simulink library "xps_library"  (Simulink 8.2)
settings: Solver=ode45  SolverMode=SingleTasking  StartTime=0.0  StopTime=10.0  RelTol=1e-3
undefined symbols (not defined in the file): sys_clk
libraries: xbsIndex_r4 x865, dspsigops x81, simulink x68, casper_library_flow_control x68, xps_library x25, casper_library_misc x4
(part 4 of 10)

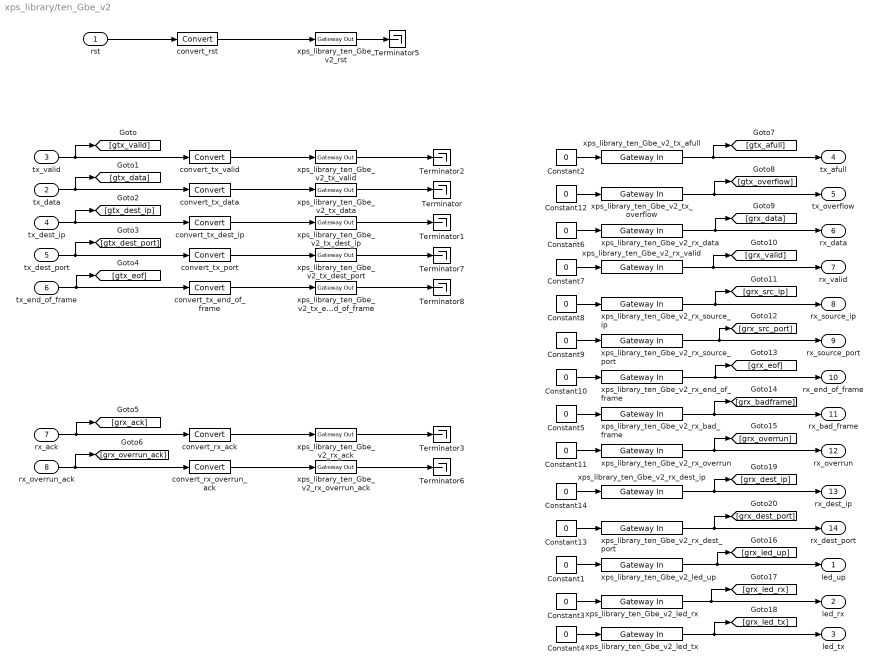
== system xps_library/ten_Gbe_v2 ==
  rst : Inport
  tx_data : Inport  Port=2
  tx_valid : Inport  Port=3
  tx_dest_ip : Inport  Port=4
  tx_dest_port : Inport  Port=5
  tx_end_of_frame : Inport  Port=6
  rx_ack : Inport  Port=7
  rx_overrun_ack : Inport  Port=8
  Constant{1..14} (14 alike) : Constant  Value=0
  Terminator{,1..3,5..8} (8 alike) : Terminator
  convert_rst : xbsIndex_r4/Convert  gui_display_data_type=Fixed-point  arith_type=Boolean  n_bits=64  bin_pt=0  float_type=Single  exp_bits=8  fraction_bits=24  quantization=Truncate  overflow=Wrap  en=off  latency=0  dbl_ovrd=off  pipeline=off  block_type=convert
      settings: xl_area=[0, 0, 0, 0, 0, 0, 0]
  convert_rx_ack : xbsIndex_r4/Convert  gui_display_data_type=Fixed-point  arith_type=Boolean  n_bits=64  bin_pt=0  float_type=Single  exp_bits=8  fraction_bits=24  quantization=Truncate  overflow=Wrap  en=off  latency=0  dbl_ovrd=off  pipeline=off  block_type=convert
      settings: xl_area=[0, 0, 0, 0, 0, 0, 0]
  convert_rx_overrun_ack : xbsIndex_r4/Convert  gui_display_data_type=Fixed-point  arith_type=Boolean  n_bits=64  bin_pt=0  float_type=Single  exp_bits=8  fraction_bits=24  quantization=Truncate  overflow=Wrap  en=off  latency=0  dbl_ovrd=off  pipeline=off  block_type=convert
      settings: xl_area=[0, 0, 0, 0, 0, 0, 0]
  convert_tx_data : xbsIndex_r4/Convert  gui_display_data_type=Fixed-point  arith_type=Unsigned  n_bits=64  bin_pt=0  float_type=Single  exp_bits=8  fraction_bits=24  quantization=Truncate  overflow=Wrap  en=off  latency=0  dbl_ovrd=off  pipeline=off  block_type=convert
      settings: xl_area=[0, 0, 0, 0, 0, 0, 0]
  convert_tx_dest_ip : xbsIndex_r4/Convert  gui_display_data_type=Fixed-point  arith_type=Unsigned  n_bits=32  bin_pt=0  float_type=Single  exp_bits=8  fraction_bits=24  quantization=Truncate  overflow=Wrap  en=off  latency=0  dbl_ovrd=off  pipeline=off  block_type=convert
      settings: xl_area=[0, 0, 0, 0, 0, 0, 0]
  convert_tx_end_of_frame : xbsIndex_r4/Convert  gui_display_data_type=Fixed-point  arith_type=Boolean  n_bits=1  bin_pt=0  float_type=Single  exp_bits=8  fraction_bits=24  quantization=Truncate  overflow=Wrap  en=off  latency=0  dbl_ovrd=off  pipeline=off  block_type=convert
      settings: xl_area=[0, 0, 0, 0, 0, 0, 0]
  convert_tx_port : xbsIndex_r4/Convert  gui_display_data_type=Fixed-point  arith_type=Unsigned  n_bits=16  bin_pt=0  float_type=Single  exp_bits=8  fraction_bits=24  quantization=Truncate  overflow=Wrap  en=off  latency=0  dbl_ovrd=off  pipeline=off  block_type=convert
      settings: xl_area=[0, 0, 0, 0, 0, 0, 0]
  convert_tx_valid : xbsIndex_r4/Convert  gui_display_data_type=Fixed-point  arith_type=Boolean  n_bits=1  bin_pt=0  float_type=Single  exp_bits=8  fraction_bits=24  quantization=Truncate  overflow=Wrap  en=off  latency=0  dbl_ovrd=off  pipeline=off  block_type=convert
      settings: xl_area=[0, 0, 0, 0, 0, 0, 0]
  xps_library_ten_Gbe_v2_led_rx : xbsIndex_r4/Gateway In  gui_display_data_type=Fixed-point  arith_type=Boolean  n_bits=1  bin_pt=0  preci_type=Single  exp_width=8  frac_width=24  quantization=Truncate  overflow=Wrap  period=1  dbl_ovrd=off  timing_constraint=None  locs_specified=off  LOCs={}  UseAsADC=off  ADCChannel='1'  inherit_from_input=off  hdl_port=on  block_type=gatewayin
      settings: infoedit="Gateway in block.  Converts inputs of type Simulink integer, double and fixed point to  Xilinx fixed point type.<P><P>Hardware notes:  In hardware these blocks become top level input ports."  xl_area=[0, 0, 0, 0, 0, 0, 0]
  xps_library_ten_Gbe_v2_led_tx : xbsIndex_r4/Gateway In  gui_display_data_type=Fixed-point  arith_type=Boolean  n_bits=1  bin_pt=0  preci_type=Single  exp_width=8  frac_width=24  quantization=Truncate  overflow=Wrap  period=1  dbl_ovrd=off  timing_constraint=None  locs_specified=off  LOCs={}  UseAsADC=off  ADCChannel='1'  inherit_from_input=off  hdl_port=on  block_type=gatewayin
      settings: infoedit="Gateway in block.  Converts inputs of type Simulink integer, double and fixed point to  Xilinx fixed point type.<P><P>Hardware notes:  In hardware these blocks become top level input ports."  xl_area=[0, 0, 0, 0, 0, 0, 0]
  xps_library_ten_Gbe_v2_led_up : xbsIndex_r4/Gateway In  gui_display_data_type=Fixed-point  arith_type=Boolean  n_bits=1  bin_pt=0  preci_type=Single  exp_width=8  frac_width=24  quantization=Truncate  overflow=Wrap  period=1  dbl_ovrd=off  timing_constraint=None  locs_specified=off  LOCs={}  UseAsADC=off  ADCChannel='1'  inherit_from_input=off  hdl_port=on  block_type=gatewayin
      settings: infoedit="Gateway in block.  Converts inputs of type Simulink integer, double and fixed point to  Xilinx fixed point type.<P><P>Hardware notes:  In hardware these blocks become top level input ports."  xl_area=[0, 0, 0, 0, 0, 0, 0]
  xps_library_ten_Gbe_v2_rst : xbsIndex_r4/Gateway Out  inherit_from_input=off  hdl_port=on  timing_constraint=None  locs_specified=off  LOCs={}  UseAsDAC=off  DACChannel='1'  block_type=gatewayout
      settings: infoedit="Gateway out block.  Converts Xilinx fixed point inputs into ouputs of type Simulink integer, double, or fixed point.<P><P>Hardware notes:  In hardware these blocks become top level output ports or are discarded, depending on how they are configured."  xl_area=[0, 0, 0, 0, 0, 0, 0]
  xps_library_ten_Gbe_v2_rx_ack : xbsIndex_r4/Gateway Out  inherit_from_input=off  hdl_port=on  timing_constraint=None  locs_specified=off  LOCs={}  UseAsDAC=off  DACChannel='1'  block_type=gatewayout
      settings: infoedit="Gateway out block.  Converts Xilinx fixed point inputs into ouputs of type Simulink integer, double, or fixed point.<P><P>Hardware notes:  In hardware these blocks become top level output ports or are discarded, depending on how they are configured."  xl_area=[0, 0, 0, 0, 0, 0, 0]
  xps_library_ten_Gbe_v2_rx_bad_frame : xbsIndex_r4/Gateway In  gui_display_data_type=Fixed-point  arith_type=Boolean  n_bits=1  bin_pt=0  preci_type=Single  exp_width=8  frac_width=24  quantization=Truncate  overflow=Wrap  period=1  dbl_ovrd=off  timing_constraint=None  locs_specified=off  LOCs={}  UseAsADC=off  ADCChannel='1'  inherit_from_input=off  hdl_port=on  block_type=gatewayin
      settings: infoedit="Gateway in block.  Converts inputs of type Simulink integer, double and fixed point to  Xilinx fixed point type.<P><P>Hardware notes:  In hardware these blocks become top level input ports."  xl_area=[0, 0, 0, 0, 0, 0, 0]
  xps_library_ten_Gbe_v2_rx_data : xbsIndex_r4/Gateway In  gui_display_data_type=Fixed-point  arith_type=Unsigned  n_bits=64  bin_pt=0  preci_type=Single  exp_width=8  frac_width=24  quantization=Truncate  overflow=Wrap  period=1  dbl_ovrd=off  timing_constraint=None  locs_specified=off  LOCs={}  UseAsADC=off  ADCChannel='1'  inherit_from_input=off  hdl_port=on  block_type=gatewayin
      settings: infoedit="Gateway in block.  Converts inputs of type Simulink integer, double and fixed point to  Xilinx fixed point type.<P><P>Hardware notes:  In hardware these blocks become top level input ports."  xl_area=[0, 0, 0, 0, 0, 0, 0]
  xps_library_ten_Gbe_v2_rx_dest_ip : xbsIndex_r4/Gateway In  gui_display_data_type=Fixed-point  arith_type=Unsigned  n_bits=32  bin_pt=0  preci_type=Single  exp_width=8  frac_width=24  quantization=Truncate  overflow=Wrap  period=1  dbl_ovrd=off  timing_constraint=None  locs_specified=off  LOCs={}  UseAsADC=off  ADCChannel='1'  inherit_from_input=off  hdl_port=on  block_type=gatewayin
      settings: xl_area=[0, 0, 0, 0, 0, 0, 0]
  xps_library_ten_Gbe_v2_rx_dest_port : xbsIndex_r4/Gateway In  gui_display_data_type=Fixed-point  arith_type=Unsigned  n_bits=16  bin_pt=0  preci_type=Single  exp_width=8  frac_width=24  quantization=Truncate  overflow=Wrap  period=1  dbl_ovrd=off  timing_constraint=None  locs_specified=off  LOCs={}  UseAsADC=off  ADCChannel='1'  inherit_from_input=off  hdl_port=on  block_type=gatewayin
      settings: xl_area=[0, 0, 0, 0, 0, 0, 0]
  xps_library_ten_Gbe_v2_rx_end_of_frame : xbsIndex_r4/Gateway In  gui_display_data_type=Fixed-point  arith_type=Boolean  n_bits=1  bin_pt=0  preci_type=Single  exp_width=8  frac_width=24  quantization=Truncate  overflow=Wrap  period=1  dbl_ovrd=off  timing_constraint=None  locs_specified=off  LOCs={}  UseAsADC=off  ADCChannel='1'  inherit_from_input=off  hdl_port=on  block_type=gatewayin
      settings: infoedit="Gateway in block.  Converts inputs of type Simulink integer, double and fixed point to  Xilinx fixed point type.<P><P>Hardware notes:  In hardware these blocks become top level input ports."  xl_area=[0, 0, 0, 0, 0, 0, 0]
  xps_library_ten_Gbe_v2_rx_overrun : xbsIndex_r4/Gateway In  gui_display_data_type=Fixed-point  arith_type=Boolean  n_bits=1  bin_pt=0  preci_type=Single  exp_width=8  frac_width=24  quantization=Truncate  overflow=Wrap  period=1  dbl_ovrd=off  timing_constraint=None  locs_specified=off  LOCs={}  UseAsADC=off  ADCChannel='1'  inherit_from_input=off  hdl_port=on  block_type=gatewayin
      settings: infoedit="Gateway in block.  Converts inputs of type Simulink integer, double and fixed point to  Xilinx fixed point type.<P><P>Hardware notes:  In hardware these blocks become top level input ports."  xl_area=[0, 0, 0, 0, 0, 0, 0]
  xps_library_ten_Gbe_v2_rx_overrun_ack : xbsIndex_r4/Gateway Out  inherit_from_input=off  hdl_port=on  timing_constraint=None  locs_specified=off  LOCs={}  UseAsDAC=off  DACChannel='1'  block_type=gatewayout
      settings: infoedit="Gateway out block.  Converts Xilinx fixed point inputs into ouputs of type Simulink integer, double, or fixed point.<P><P>Hardware notes:  In hardware these blocks become top level output ports or are discarded, depending on how they are configured."  xl_area=[0, 0, 0, 0, 0, 0, 0]
  xps_library_ten_Gbe_v2_rx_source_ip : xbsIndex_r4/Gateway In  gui_display_data_type=Fixed-point  arith_type=Unsigned  n_bits=32  bin_pt=0  preci_type=Single  exp_width=8  frac_width=24  quantization=Truncate  overflow=Wrap  period=1  dbl_ovrd=off  timing_constraint=None  locs_specified=off  LOCs={}  UseAsADC=off  ADCChannel='1'  inherit_from_input=off  hdl_port=on  block_type=gatewayin
      settings: infoedit="Gateway in block.  Converts inputs of type Simulink integer, double and fixed point to  Xilinx fixed point type.<P><P>Hardware notes:  In hardware these blocks become top level input ports."  xl_area=[0, 0, 0, 0, 0, 0, 0]
  xps_library_ten_Gbe_v2_rx_source_port : xbsIndex_r4/Gateway In  gui_display_data_type=Fixed-point  arith_type=Unsigned  n_bits=16  bin_pt=0  preci_type=Single  exp_width=8  frac_width=24  quantization=Truncate  overflow=Wrap  period=1  dbl_ovrd=off  timing_constraint=None  locs_specified=off  LOCs={}  UseAsADC=off  ADCChannel='1'  inherit_from_input=off  hdl_port=on  block_type=gatewayin
      settings: infoedit="Gateway in block.  Converts inputs of type Simulink integer, double and fixed point to  Xilinx fixed point type.<P><P>Hardware notes:  In hardware these blocks become top level input ports."  xl_area=[0, 0, 0, 0, 0, 0, 0]
  xps_library_ten_Gbe_v2_rx_valid : xbsIndex_r4/Gateway In  gui_display_data_type=Fixed-point  arith_type=Boolean  n_bits=1  bin_pt=0  preci_type=Single  exp_width=8  frac_width=24  quantization=Truncate  overflow=Wrap  period=1  dbl_ovrd=off  timing_constraint=None  locs_specified=off  LOCs={}  UseAsADC=off  ADCChannel='1'  inherit_from_input=off  hdl_port=on  block_type=gatewayin
      settings: infoedit="Gateway in block.  Converts inputs of type Simulink integer, double and fixed point to  Xilinx fixed point type.<P><P>Hardware notes:  In hardware these blocks become top level input ports."  xl_area=[0, 0, 0, 0, 0, 0, 0]
  xps_library_ten_Gbe_v2_tx_afull : xbsIndex_r4/Gateway In  gui_display_data_type=Fixed-point  arith_type=Boolean  n_bits=1  bin_pt=0  preci_type=Single  exp_width=8  frac_width=24  quantization=Truncate  overflow=Wrap  period=1  dbl_ovrd=off  timing_constraint=None  locs_specified=off  LOCs={}  UseAsADC=off  ADCChannel='1'  inherit_from_input=off  hdl_port=on  block_type=gatewayin
      settings: infoedit="Gateway in block.  Converts inputs of type Simulink integer, double and fixed point to  Xilinx fixed point type.<P><P>Hardware notes:  In hardware these blocks become top level input ports."  xl_area=[0, 0, 0, 0, 0, 0, 0]
  xps_library_ten_Gbe_v2_tx_data : xbsIndex_r4/Gateway Out  inherit_from_input=off  hdl_port=on  timing_constraint=None  locs_specified=off  LOCs={}  UseAsDAC=off  DACChannel='1'  block_type=gatewayout
      settings: infoedit="Gateway out block.  Converts Xilinx fixed point inputs into ouputs of type Simulink integer, double, or fixed point.<P><P>Hardware notes:  In hardware these blocks become top level output ports or are discarded, depending on how they are configured."  xl_area=[0, 0, 0, 0, 0, 0, 0]
  xps_library_ten_Gbe_v2_tx_dest_ip : xbsIndex_r4/Gateway Out  inherit_from_input=off  hdl_port=on  timing_constraint=None  locs_specified=off  LOCs={}  UseAsDAC=off  DACChannel='1'  block_type=gatewayout
      settings: infoedit="Gateway out block.  Converts Xilinx fixed point inputs into ouputs of type Simulink integer, double, or fixed point.<P><P>Hardware notes:  In hardware these blocks become top level output ports or are discarded, depending on how they are configured."  xl_area=[0, 0, 0, 0, 0, 0, 0]
  xps_library_ten_Gbe_v2_tx_dest_port : xbsIndex_r4/Gateway Out  inherit_from_input=off  hdl_port=on  timing_constraint=None  locs_specified=off  LOCs={}  UseAsDAC=off  DACChannel='1'  block_type=gatewayout
      settings: infoedit="Gateway out block.  Converts Xilinx fixed point inputs into ouputs of type Simulink integer, double, or fixed point.<P><P>Hardware notes:  In hardware these blocks become top level output ports or are discarded, depending on how they are configured."  xl_area=[0, 0, 0, 0, 0, 0, 0]
  xps_library_ten_Gbe_v2_tx_end_of_frame : xbsIndex_r4/Gateway Out  inherit_from_input=off  hdl_port=on  timing_constraint=None  locs_specified=off  LOCs={}  UseAsDAC=off  DACChannel='1'  block_type=gatewayout
      settings: infoedit="Gateway out block.  Converts Xilinx fixed point inputs into ouputs of type Simulink integer, double, or fixed point.<P><P>Hardware notes:  In hardware these blocks become top level output ports or are discarded, depending on how they are configured."  xl_area=[0, 0, 0, 0, 0, 0, 0]
  xps_library_ten_Gbe_v2_tx_overflow : xbsIndex_r4/Gateway In  gui_display_data_type=Fixed-point  arith_type=Boolean  n_bits=1  bin_pt=0  preci_type=Single  exp_width=8  frac_width=24  quantization=Truncate  overflow=Wrap  period=1  dbl_ovrd=off  timing_constraint=None  locs_specified=off  LOCs={}  UseAsADC=off  ADCChannel='1'  inherit_from_input=off  hdl_port=on  block_type=gatewayin
      settings: infoedit="Gateway in block.  Converts inputs of type Simulink integer, double and fixed point to  Xilinx fixed point type.<P><P>Hardware notes:  In hardware these blocks become top level input ports."  xl_area=[0, 0, 0, 0, 0, 0, 0]
  xps_library_ten_Gbe_v2_tx_valid : xbsIndex_r4/Gateway Out  inherit_from_input=off  hdl_port=on  timing_constraint=None  locs_specified=off  LOCs={}  UseAsDAC=off  DACChannel='1'  block_type=gatewayout
      settings: infoedit="Gateway out block.  Converts Xilinx fixed point inputs into ouputs of type Simulink integer, double, or fixed point.<P><P>Hardware notes:  In hardware these blocks become top level output ports or are discarded, depending on how they are configured."  xl_area=[0, 0, 0, 0, 0, 0, 0]
  led_up : Outport
  led_rx : Outport  Port=2
  led_tx : Outport  Port=3
  tx_afull : Outport  Port=4
  tx_overflow : Outport  Port=5
  rx_data : Outport  Port=6
  rx_valid : Outport  Port=7
  rx_source_ip : Outport  Port=8
  rx_source_port : Outport  Port=9
  rx_end_of_frame : Outport  Port=10
  rx_bad_frame : Outport  Port=11
  rx_overrun : Outport  Port=12
  rx_dest_ip : Outport  Port=13
  rx_dest_port : Outport  Port=14
  wires:
  xps_library_ten_Gbe_v2_tx_overflow/1 -> [gtx_overflow], tx_overflow/1
  Constant12/1 -> xps_library_ten_Gbe_v2_tx_overflow/1
  rx_overrun_ack/1 -> [grx_overrun_ack], convert_rx_overrun_ack/1
  convert_rx_overrun_ack/1 -> xps_library_ten_Gbe_v2_rx_overrun_ack/1
  xps_library_ten_Gbe_v2_rx_overrun_ack/1 -> Terminator6/1
  Constant11/1 -> xps_library_ten_Gbe_v2_rx_overrun/1
  xps_library_ten_Gbe_v2_rx_overrun/1 -> [grx_overrun], rx_overrun/1
  Constant5/1 -> xps_library_ten_Gbe_v2_rx_bad_frame/1
  xps_library_ten_Gbe_v2_rx_bad_frame/1 -> [grx_badframe], rx_bad_frame/1
  rx_ack/1 -> [grx_ack], convert_rx_ack/1
  convert_rx_ack/1 -> xps_library_ten_Gbe_v2_rx_ack/1
  xps_library_ten_Gbe_v2_rx_data/1 -> [grx_data], rx_data/1
  tx_data/1 -> [gtx_data], convert_tx_data/1
  convert_tx_data/1 -> xps_library_ten_Gbe_v2_tx_data/1
  tx_dest_ip/1 -> [gtx_dest_ip], convert_tx_dest_ip/1
  convert_tx_dest_ip/1 -> xps_library_ten_Gbe_v2_tx_dest_ip/1
  tx_valid/1 -> [gtx_valid], convert_tx_valid/1
  convert_tx_valid/1 -> xps_library_ten_Gbe_v2_tx_valid/1
  xps_library_ten_Gbe_v2_tx_afull/1 -> [gtx_afull], tx_afull/1
  xps_library_ten_Gbe_v2_tx_data/1 -> Terminator/1
  xps_library_ten_Gbe_v2_tx_dest_ip/1 -> Terminator1/1
  xps_library_ten_Gbe_v2_tx_valid/1 -> Terminator2/1
  Constant2/1 -> xps_library_ten_Gbe_v2_tx_afull/1
  Constant6/1 -> xps_library_ten_Gbe_v2_rx_data/1
  xps_library_ten_Gbe_v2_rx_ack/1 -> Terminator3/1
  Constant7/1 -> xps_library_ten_Gbe_v2_rx_valid/1
  xps_library_ten_Gbe_v2_rx_valid/1 -> [grx_valid], rx_valid/1
  rst/1 -> convert_rst/1
  convert_rst/1 -> xps_library_ten_Gbe_v2_rst/1
  xps_library_ten_Gbe_v2_rst/1 -> Terminator5/1
  tx_dest_port/1 -> [gtx_dest_port], convert_tx_port/1
  convert_tx_port/1 -> xps_library_ten_Gbe_v2_tx_dest_port/1
  xps_library_ten_Gbe_v2_tx_dest_port/1 -> Terminator7/1
  tx_end_of_frame/1 -> [gtx_eof], convert_tx_end_of_frame/1
  convert_tx_end_of_frame/1 -> xps_library_ten_Gbe_v2_tx_end_of_frame/1
  xps_library_ten_Gbe_v2_tx_end_of_frame/1 -> Terminator8/1
  xps_library_ten_Gbe_v2_rx_source_ip/1 -> [grx_src_ip], rx_source_ip/1
  Constant8/1 -> xps_library_ten_Gbe_v2_rx_source_ip/1
  Constant9/1 -> xps_library_ten_Gbe_v2_rx_source_port/1
  xps_library_ten_Gbe_v2_rx_source_port/1 -> [grx_src_port], rx_source_port/1
  Constant10/1 -> xps_library_ten_Gbe_v2_rx_end_of_frame/1
  xps_library_ten_Gbe_v2_rx_end_of_frame/1 -> [grx_eof], rx_end_of_frame/1
  Constant1/1 -> xps_library_ten_Gbe_v2_led_up/1
  xps_library_ten_Gbe_v2_led_up/1 -> [grx_led_up], led_up/1
  Constant3/1 -> xps_library_ten_Gbe_v2_led_rx/1
  xps_library_ten_Gbe_v2_led_rx/1 -> [grx_led_rx], led_rx/1
  Constant4/1 -> xps_library_ten_Gbe_v2_led_tx/1
  xps_library_ten_Gbe_v2_led_tx/1 -> [grx_led_tx], led_tx/1
  Constant13/1 -> xps_library_ten_Gbe_v2_rx_dest_port/1
  xps_library_ten_Gbe_v2_rx_dest_port/1 -> rx_dest_port/1, [grx_dest_port]
  Constant14/1 -> xps_library_ten_Gbe_v2_rx_dest_ip/1
  xps_library_ten_Gbe_v2_rx_dest_ip/1 -> rx_dest_ip/1, [grx_dest_ip]

== system xps_library/ucf ==

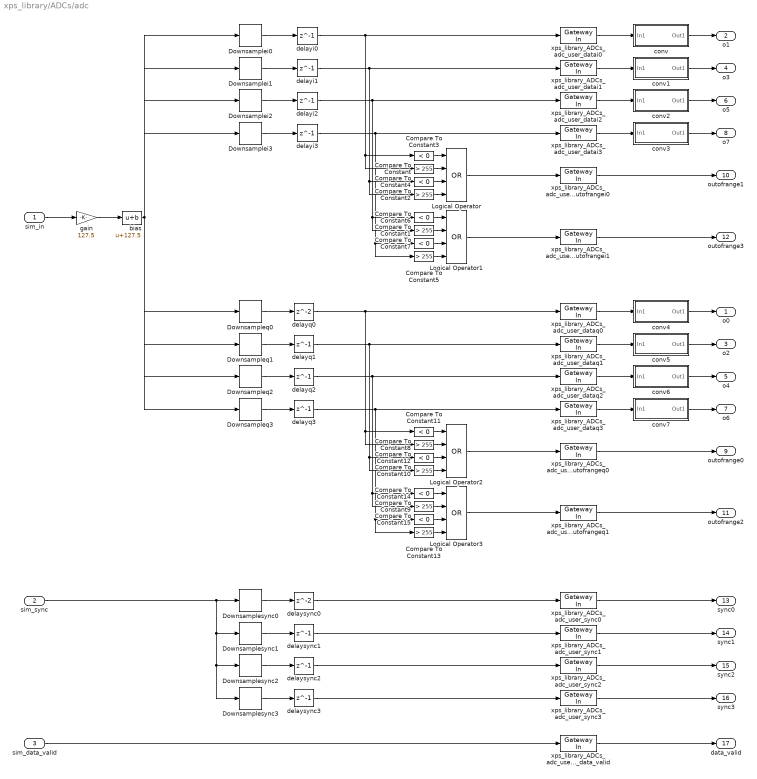
== system xps_library/ADCs/adc ==
  sim_in : Inport  SampleTime=sample_period/8
  sim_sync : Inport  Port=2  SampleTime=sample_period/8
  sim_data_valid : Inport  Port=3  SampleTime=sample_period/4
  Compare To Constant{,1..2,5,8..10,13} (8 alike) : simulink/Logic and Bit Operations/Compare To Constant  relop=>  const=255  OutDataTypeStr=boolean  ZeroCross=off
  Compare To Constant{3..4,6..7,11..12,14..15} (8 alike) : simulink/Logic and Bit Operations/Compare To Constant  relop=<  const=0  OutDataTypeStr=boolean  ZeroCross=off
  Downsamplei0 : dspsigops/Downsample  N=8  phase=1  RateOptions=Allow multirate processing  smode=Allow multirate  fmode=Maintain input frame size  ic=0
  Downsamplei1 : dspsigops/Downsample  N=8  phase=3  RateOptions=Allow multirate processing  smode=Allow multirate  fmode=Maintain input frame size  ic=0
  Downsamplei2 : dspsigops/Downsample  N=8  phase=5  RateOptions=Allow multirate processing  smode=Allow multirate  fmode=Maintain input frame size  ic=0
  Downsamplei3 : dspsigops/Downsample  N=8  phase=7  RateOptions=Allow multirate processing  smode=Allow multirate  fmode=Maintain input frame size  ic=0
  Downsampleq0 : dspsigops/Downsample  N=8  phase=0  RateOptions=Allow multirate processing  smode=Allow multirate  fmode=Maintain input frame size  ic=0
  Downsampleq1 : dspsigops/Downsample  N=8  phase=2  RateOptions=Allow multirate processing  smode=Allow multirate  fmode=Maintain input frame size  ic=0
  Downsampleq2 : dspsigops/Downsample  N=8  phase=4  RateOptions=Allow multirate processing  smode=Allow multirate  fmode=Maintain input frame size  ic=0
  Downsampleq3 : dspsigops/Downsample  N=8  phase=6  RateOptions=Allow multirate processing  smode=Allow multirate  fmode=Maintain input frame size  ic=0
  Downsamplesync0 : dspsigops/Downsample  N=8  phase=0  RateOptions=Allow multirate processing  smode=Allow multirate  fmode=Maintain input frame size  ic=0
  Downsamplesync1 : dspsigops/Downsample  N=8  phase=2  RateOptions=Allow multirate processing  smode=Allow multirate  fmode=Maintain input frame size  ic=0
  Downsamplesync2 : dspsigops/Downsample  N=8  phase=4  RateOptions=Allow multirate processing  smode=Allow multirate  fmode=Maintain input frame size  ic=0
  Downsamplesync3 : dspsigops/Downsample  N=8  phase=6  RateOptions=Allow multirate processing  smode=Allow multirate  fmode=Maintain input frame size  ic=0
  Logical Operator{,1..3} (4 alike) : Logic  Operator=OR  Inputs=4  AllPortsSameDT=off  OutDataTypeStr=boolean
  bias : Bias  Bias=127.5  SaturateOnIntegerOverflow=on
  conv : Subsystem
  conv1 : Subsystem
  conv2 : Subsystem
  conv3 : Subsystem
  conv4 : Subsystem
  conv5 : Subsystem
  conv6 : Subsystem
  conv7 : Subsystem
  delayi{0..3} (4 alike) : Delay  DelayLength=1  InputProcessing=Inherited
  delayq0 : Delay  InputProcessing=Inherited
  delayq1 : Delay  DelayLength=1  InputProcessing=Inherited
  delayq2 : Delay  DelayLength=1  InputProcessing=Inherited
  delayq3 : Delay  DelayLength=1  InputProcessing=Inherited
  delaysync0 : Delay  InputProcessing=Inherited
  delaysync1 : Delay  DelayLength=1  InputProcessing=Inherited
  delaysync2 : Delay  DelayLength=1  InputProcessing=Inherited
  delaysync3 : Delay  DelayLength=1  InputProcessing=Inherited
  gain : Gain  Gain=127.5  SaturateOnIntegerOverflow=on  OutDataTypeStr=Inherit: Same as input  ParamDataTypeStr=Inherit: Same as input
  xps_library_ADCs_adc_user_data_valid : xbsIndex_r4/Gateway In  gui_display_data_type=Fixed-point  arith_type=Boolean  n_bits=8  bin_pt=0  preci_type=Single  exp_width=8  frac_width=24  quantization="Round  (unbiased: +/- Inf)"  overflow=Saturate  period=sample_period  dbl_ovrd=off  timing_constraint=None  locs_specified=off  LOCs={}  UseAsADC=off  ADCChannel='1'  inherit_from_input=off  hdl_port=on  block_type=gatewayin
      settings: infoedit="Gateway in block.  Converts inputs of type Simulink integer, double and fixed point to  Xilinx fixed point type.<P><P>Hardware notes:  In hardware these blocks become top level input ports."  xl_area=[0 0 0 0 8 0 0]  block_version=8.2.02
  xps_library_ADCs_adc_user_datai{0..3} (4 alike) : xbsIndex_r4/Gateway In  gui_display_data_type=Fixed-point  arith_type=Unsigned  n_bits=8  bin_pt=0  preci_type=Single  exp_width=8  frac_width=24  quantization="Round  (unbiased: +/- Inf)"  overflow=Saturate  period=sample_period  dbl_ovrd=off  timing_constraint=None  locs_specified=off  LOCs={}  UseAsADC=off  ADCChannel='1'  inherit_from_input=off  hdl_port=on  block_type=gatewayin
      settings: infoedit="Gateway in block.  Converts inputs of type Simulink integer, double and fixed point to  Xilinx fixed point type.<P><P>Hardware notes:  In hardware these blocks become top level input ports."  xl_area=[0 0 0 0 8 0 0]  block_version=8.2.02
  xps_library_ADCs_adc_user_dataq{0..3} (4 alike) : xbsIndex_r4/Gateway In  gui_display_data_type=Fixed-point  arith_type=Unsigned  n_bits=8  bin_pt=0  preci_type=Single  exp_width=8  frac_width=24  quantization="Round  (unbiased: +/- Inf)"  overflow=Saturate  period=sample_period  dbl_ovrd=off  timing_constraint=None  locs_specified=off  LOCs={}  UseAsADC=off  ADCChannel='1'  inherit_from_input=off  hdl_port=on  block_type=gatewayin
      settings: infoedit="Gateway in block.  Converts inputs of type Simulink integer, double and fixed point to  Xilinx fixed point type.<P><P>Hardware notes:  In hardware these blocks become top level input ports."  xl_area=[0 0 0 0 8 0 0]  block_version=8.2.02
  xps_library_ADCs_adc_user_outofrangei0 : xbsIndex_r4/Gateway In  gui_display_data_type=Fixed-point  arith_type=Boolean  n_bits=8  bin_pt=0  preci_type=Single  exp_width=8  frac_width=24  quantization="Round  (unbiased: +/- Inf)"  overflow=Saturate  period=sample_period  dbl_ovrd=off  timing_constraint=None  locs_specified=off  LOCs={}  UseAsADC=off  ADCChannel='1'  inherit_from_input=off  hdl_port=on  block_type=gatewayin
      settings: infoedit="Gateway in block.  Converts inputs of type Simulink integer, double and fixed point to  Xilinx fixed point type.<P><P>Hardware notes:  In hardware these blocks become top level input ports."  xl_area=[0 0 0 0 8 0 0]  block_version=8.2.02
  xps_library_ADCs_adc_user_outofrangei1 : xbsIndex_r4/Gateway In  gui_display_data_type=Fixed-point  arith_type=Boolean  n_bits=8  bin_pt=0  preci_type=Single  exp_width=8  frac_width=24  quantization="Round  (unbiased: +/- Inf)"  overflow=Saturate  period=sample_period  dbl_ovrd=off  timing_constraint=None  locs_specified=off  LOCs={}  UseAsADC=off  ADCChannel='1'  inherit_from_input=off  hdl_port=on  block_type=gatewayin
      settings: infoedit="Gateway in block.  Converts inputs of type Simulink integer, double and fixed point to  Xilinx fixed point type.<P><P>Hardware notes:  In hardware these blocks become top level input ports."  xl_area=[0 0 0 0 8 0 0]  block_version=8.2.02
  xps_library_ADCs_adc_user_outofrangeq0 : xbsIndex_r4/Gateway In  gui_display_data_type=Fixed-point  arith_type=Boolean  n_bits=8  bin_pt=0  preci_type=Single  exp_width=8  frac_width=24  quantization="Round  (unbiased: +/- Inf)"  overflow=Saturate  period=sample_period  dbl_ovrd=off  timing_constraint=None  locs_specified=off  LOCs={}  UseAsADC=off  ADCChannel='1'  inherit_from_input=off  hdl_port=on  block_type=gatewayin
      settings: infoedit="Gateway in block.  Converts inputs of type Simulink integer, double and fixed point to  Xilinx fixed point type.<P><P>Hardware notes:  In hardware these blocks become top level input ports."  xl_area=[0 0 0 0 8 0 0]  block_version=8.2.02
  xps_library_ADCs_adc_user_outofrangeq1 : xbsIndex_r4/Gateway In  gui_display_data_type=Fixed-point  arith_type=Boolean  n_bits=8  bin_pt=0  preci_type=Single  exp_width=8  frac_width=24  quantization="Round  (unbiased: +/- Inf)"  overflow=Saturate  period=sample_period  dbl_ovrd=off  timing_constraint=None  locs_specified=off  LOCs={}  UseAsADC=off  ADCChannel='1'  inherit_from_input=off  hdl_port=on  block_type=gatewayin
      settings: infoedit="Gateway in block.  Converts inputs of type Simulink integer, double and fixed point to  Xilinx fixed point type.<P><P>Hardware notes:  In hardware these blocks become top level input ports."  xl_area=[0 0 0 0 8 0 0]  block_version=8.2.02
  xps_library_ADCs_adc_user_sync{0..3} (4 alike) : xbsIndex_r4/Gateway In  gui_display_data_type=Fixed-point  arith_type=Boolean  n_bits=8  bin_pt=0  preci_type=Single  exp_width=8  frac_width=24  quantization="Round  (unbiased: +/- Inf)"  overflow=Saturate  period=sample_period  dbl_ovrd=off  timing_constraint=None  locs_specified=off  LOCs={}  UseAsADC=off  ADCChannel='1'  inherit_from_input=off  hdl_port=on  block_type=gatewayin
      settings: infoedit="Gateway in block.  Converts inputs of type Simulink integer, double and fixed point to  Xilinx fixed point type.<P><P>Hardware notes:  In hardware these blocks become top level input ports."  xl_area=[0 0 0 0 8 0 0]  block_version=8.2.02
  o0 : Outport
  o1 : Outport  Port=2
  o2 : Outport  Port=3
  o3 : Outport  Port=4
  o4 : Outport  Port=5
  o5 : Outport  Port=6
  o6 : Outport  Port=7
  o7 : Outport  Port=8
  outofrange0 : Outport  Port=9
  outofrange1 : Outport  Port=10
  outofrange2 : Outport  Port=11
  outofrange3 : Outport  Port=12
  sync0 : Outport  Port=13
  sync1 : Outport  Port=14
  sync2 : Outport  Port=15
  sync3 : Outport  Port=16
  data_valid : Outport  Port=17
  wires:
  bias/1 -> Downsampleq3/1, Downsampleq2/1, Downsampleq1/1, Downsampleq0/1, Downsamplei3/1, Downsamplei2/1, Downsamplei1/1, Downsamplei0/1
  gain/1 -> bias/1
  sim_in/1 -> gain/1
  xps_library_ADCs_adc_user_datai0/1 -> conv/1(In1)
  sim_data_valid/1 -> xps_library_ADCs_adc_user_data_valid/1
  xps_library_ADCs_adc_user_data_valid/1 -> data_valid/1
  xps_library_ADCs_adc_user_sync3/1 -> sync3/1
  xps_library_ADCs_adc_user_sync2/1 -> sync2/1
  delaysync3/1 -> xps_library_ADCs_adc_user_sync3/1
  delaysync2/1 -> xps_library_ADCs_adc_user_sync2/1
  Downsamplesync3/1 -> delaysync3/1
  Downsamplesync2/1 -> delaysync2/1
  xps_library_ADCs_adc_user_sync1/1 -> sync1/1
  delaysync0/1 -> xps_library_ADCs_adc_user_sync0/1
  Downsamplesync1/1 -> delaysync1/1
  Downsamplesync0/1 -> delaysync0/1
  sim_sync/1 -> Downsamplesync3/1, Downsamplesync2/1, Downsamplesync1/1, Downsamplesync0/1
  Logical Operator3/1 -> xps_library_ADCs_adc_user_outofrangeq1/1
  Compare To Constant13/1 -> Logical Operator3/4
  Compare To Constant15/1 -> Logical Operator3/3
  Compare To Constant9/1 -> Logical Operator3/2
  Compare To Constant14/1 -> Logical Operator3/1
  Logical Operator2/1 -> xps_library_ADCs_adc_user_outofrangeq0/1
  Compare To Constant10/1 -> Logical Operator2/4
  Compare To Constant12/1 -> Logical Operator2/3
  Compare To Constant8/1 -> Logical Operator2/2
  Compare To Constant11/1 -> Logical Operator2/1
  xps_library_ADCs_adc_user_outofrangeq1/1 -> outofrange2/1
  xps_library_ADCs_adc_user_outofrangeq0/1 -> outofrange0/1
  Logical Operator1/1 -> xps_library_ADCs_adc_user_outofrangei1/1
  Compare To Constant5/1 -> Logical Operator1/4
  Compare To Constant7/1 -> Logical Operator1/3
  Compare To Constant1/1 -> Logical Operator1/2
  Compare To Constant6/1 -> Logical Operator1/1
  Logical Operator/1 -> xps_library_ADCs_adc_user_outofrangei0/1
  Compare To Constant2/1 -> Logical Operator/4
  Compare To Constant4/1 -> Logical Operator/3
  Compare To Constant/1 -> Logical Operator/2
  Compare To Constant3/1 -> Logical Operator/1
  xps_library_ADCs_adc_user_outofrangei1/1 -> outofrange3/1
  delayq0/1 -> Compare To Constant8/1, Compare To Constant11/1, xps_library_ADCs_adc_user_dataq0/1
  Downsampleq0/1 -> delayq0/1
  delayi0/1 -> Compare To Constant3/1, Compare To Constant/1, xps_library_ADCs_adc_user_datai0/1
  Downsamplei1/1 -> delayi1/1
  Downsamplei2/1 -> delayi2/1
  Downsamplei3/1 -> delayi3/1
  Downsampleq1/1 -> delayq1/1
  Downsampleq2/1 -> delayq2/1
  Downsampleq3/1 -> delayq3/1
  xps_library_ADCs_adc_user_datai1/1 -> conv1/1(In1)
  xps_library_ADCs_adc_user_datai2/1 -> conv2/1(In1)
  xps_library_ADCs_adc_user_datai3/1 -> conv3/1(In1)
  xps_library_ADCs_adc_user_outofrangei0/1 -> outofrange1/1
  xps_library_ADCs_adc_user_sync0/1 -> sync0/1
  conv/1(Out1) -> o1/1
  conv1/1(Out1) -> o3/1
  conv2/1(Out1) -> o5/1
  conv3/1(Out1) -> o7/1
  xps_library_ADCs_adc_user_dataq0/1 -> conv4/1(In1)
  conv4/1(Out1) -> o0/1
  xps_library_ADCs_adc_user_dataq1/1 -> conv5/1(In1)
  conv5/1(Out1) -> o2/1
  xps_library_ADCs_adc_user_dataq2/1 -> conv6/1(In1)
  conv6/1(Out1) -> o4/1
  xps_library_ADCs_adc_user_dataq3/1 -> conv7/1(In1)
  conv7/1(Out1) -> o6/1
  Downsamplei0/1 -> delayi0/1
  delayi1/1 -> Compare To Constant4/1, Compare To Constant2/1, xps_library_ADCs_adc_user_datai1/1
  delayi2/1 -> Compare To Constant1/1, Compare To Constant6/1, xps_library_ADCs_adc_user_datai2/1
  delayi3/1 -> Compare To Constant5/1, Compare To Constant7/1, xps_library_ADCs_adc_user_datai3/1
  delayq1/1 -> Compare To Constant10/1, Compare To Constant12/1, xps_library_ADCs_adc_user_dataq1/1
  delayq2/1 -> Compare To Constant9/1, Compare To Constant14/1, xps_library_ADCs_adc_user_dataq2/1
  delayq3/1 -> Compare To Constant13/1, Compare To Constant15/1, xps_library_ADCs_adc_user_dataq3/1
  delaysync1/1 -> xps_library_ADCs_adc_user_sync1/1

== system xps_library/ADCs/adc083000_ctrl ==
  conf : Inport
  sdata_bus : Inport  Port=2
  Convert : xbsIndex_r4/Convert  gui_display_data_type=Fixed-point  arith_type=Unsigned  n_bits=3  bin_pt=0  float_type=Single  exp_bits=8  fraction_bits=24  quantization=Truncate  overflow=Wrap  en=off  latency=2  dbl_ovrd=off  pipeline=off  block_type=convert
      settings: block_version=11.4
  Convert1 : xbsIndex_r4/Convert  gui_display_data_type=Fixed-point  arith_type=Unsigned  n_bits=32  bin_pt=0  float_type=Single  exp_bits=8  fraction_bits=24  quantization=Truncate  overflow=Wrap  en=off  latency=2  dbl_ovrd=off  pipeline=off  block_type=convert
      settings: block_version=11.4
  Slice : xbsIndex_r4/Slice  nbits=3  boolean_output=off  mode=Lower Bit Location + Width  bit1=0  base1=MSB of Input  bit0=0  base0=LSB of Input  dbl_ovrd=off  block_type=slice
  Terminator : Terminator
  Terminator1 : Terminator
  xps_library_ADCs_adc083000_ctrl_conf : xbsIndex_r4/Gateway Out  inherit_from_input=off  hdl_port=on  timing_constraint=None  locs_specified=off  LOCs={}  UseAsDAC=off  DACChannel='1'  block_type=gatewayout
      settings: infoedit="Gateway out block.  Converts Xilinx fixed point inputs into ouputs of type Simulink integer, double, or fixed point.<br><br>Hardware notes:  In hardware these blocks become top level output ports or are discarded, depending on how they are configured."  block_version=11.4
  xps_library_ADCs_adc083000_ctrl_sdata_bus : xbsIndex_r4/Gateway Out  inherit_from_input=off  hdl_port=on  timing_constraint=None  locs_specified=off  LOCs={}  UseAsDAC=off  DACChannel='1'  block_type=gatewayout
      settings: infoedit="Gateway out block.  Converts Xilinx fixed point inputs into ouputs of type Simulink integer, double, or fixed point.<br><br>Hardware notes:  In hardware these blocks become top level output ports or are discarded, depending on how they are configured."  block_version=11.4
  wires:
  xps_library_ADCs_adc083000_ctrl_sdata_bus/1 -> Terminator1/1
  xps_library_ADCs_adc083000_ctrl_conf/1 -> Terminator/1
  Convert1/1 -> xps_library_ADCs_adc083000_ctrl_sdata_bus/1
  Slice/1 -> Convert/1
  conf/1 -> Slice/1
  Convert/1 -> xps_library_ADCs_adc083000_ctrl_conf/1
  sdata_bus/1 -> Convert1/1

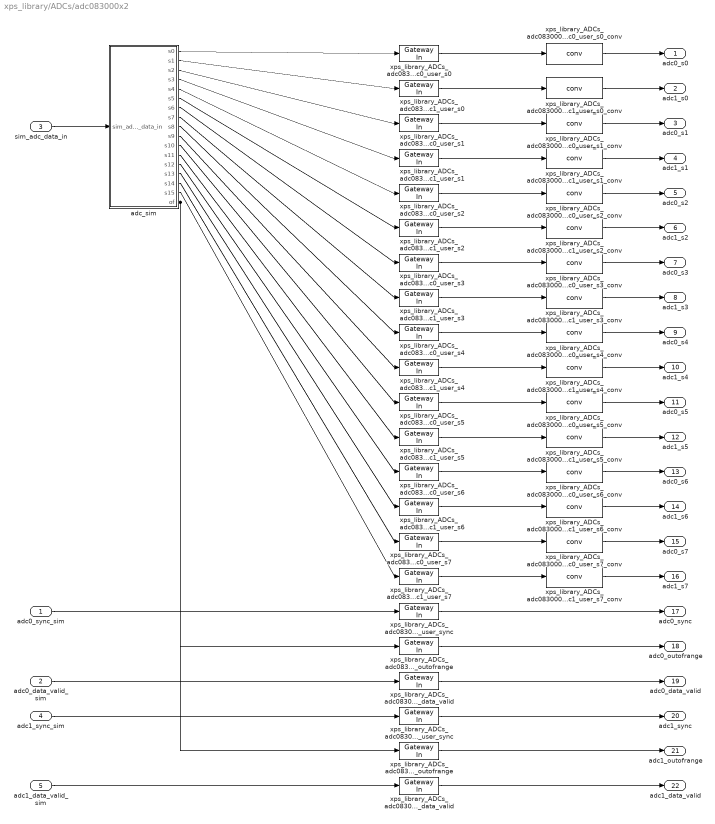
== system xps_library/ADCs/adc083000x2 ==
  adc0_sync_sim : Inport
  adc0_data_valid_sim : Inport  Port=2
  sim_adc_data_in : Inport  Port=3
  adc1_sync_sim : Inport  Port=4
  adc1_data_valid_sim : Inport  Port=5
  adc_sim : Subsystem  AncestorBlock=xps_library/ADCs/adc_sim  mask(adc_sim){nStreams=16, bit_width=8}
      mask prompts: nStreams "Number of Output Streams"; bit_width "Sample Bit Width"
      mask help:
      | This block simulates the behavior of a demuxed ADC, which takes
      | as input a waveform and returns digital samples in parallel at
      | a slower rate.
      |
      | This block is used to simulate the behavior
      mask init:
      | adc_sim_init(gcb, ...
      |     'nStreams', nStreams, ...
      |     'bit_width', bit_width);
  xps_library_ADCs_adc083000x2_adc0_user_data_valid : xbsIndex_r4/Gateway In  gui_display_data_type=Fixed-point  arith_type=Unsigned  n_bits=1  bin_pt=0  preci_type=Single  exp_width=8  frac_width=24  quantization="Round  (unbiased: +/- Inf)"  overflow=Saturate  period=1  dbl_ovrd=off  timing_constraint=None  locs_specified=off  LOCs={}  UseAsADC=off  ADCChannel='1'  inherit_from_input=off  hdl_port=on  block_type=gatewayin
  xps_library_ADCs_adc083000x2_adc0_user_outofrange : xbsIndex_r4/Gateway In  gui_display_data_type=Fixed-point  arith_type=Unsigned  n_bits=4  bin_pt=0  preci_type=Single  exp_width=8  frac_width=24  quantization="Round  (unbiased: +/- Inf)"  overflow=Saturate  period=1  dbl_ovrd=off  timing_constraint=None  locs_specified=off  LOCs={}  UseAsADC=off  ADCChannel='1'  inherit_from_input=off  hdl_port=on  block_type=gatewayin
  xps_library_ADCs_adc083000x2_adc0_user_s{0..7} (8 alike) : xbsIndex_r4/Gateway In  gui_display_data_type=Fixed-point  arith_type=Unsigned  n_bits=8  bin_pt=0  preci_type=Single  exp_width=8  frac_width=24  quantization="Round  (unbiased: +/- Inf)"  overflow=Saturate  period=1  dbl_ovrd=off  timing_constraint=None  locs_specified=off  LOCs={}  UseAsADC=off  ADCChannel='1'  inherit_from_input=off  hdl_port=on  block_type=gatewayin
  xps_library_ADCs_adc083000x2_adc0_user_s0_conv : xps_library/ADCs/conv  bit_width=8
  xps_library_ADCs_adc083000x2_adc0_user_s1_conv : xps_library/ADCs/conv  bit_width=8
  xps_library_ADCs_adc083000x2_adc0_user_s2_conv : xps_library/ADCs/conv  bit_width=8
  xps_library_ADCs_adc083000x2_adc0_user_s3_conv : xps_library/ADCs/conv  bit_width=8
  xps_library_ADCs_adc083000x2_adc0_user_s4_conv : xps_library/ADCs/conv  bit_width=8
  xps_library_ADCs_adc083000x2_adc0_user_s5_conv : xps_library/ADCs/conv  bit_width=8
  xps_library_ADCs_adc083000x2_adc0_user_s6_conv : xps_library/ADCs/conv  bit_width=8
  xps_library_ADCs_adc083000x2_adc0_user_s7_conv : xps_library/ADCs/conv  bit_width=8
  xps_library_ADCs_adc083000x2_adc0_user_sync : xbsIndex_r4/Gateway In  gui_display_data_type=Fixed-point  arith_type=Unsigned  n_bits=4  bin_pt=0  preci_type=Single  exp_width=8  frac_width=24  quantization="Round  (unbiased: +/- Inf)"  overflow=Saturate  period=1  dbl_ovrd=off  timing_constraint=None  locs_specified=off  LOCs={}  UseAsADC=off  ADCChannel='1'  inherit_from_input=off  hdl_port=on  block_type=gatewayin
  xps_library_ADCs_adc083000x2_adc1_user_data_valid : xbsIndex_r4/Gateway In  gui_display_data_type=Fixed-point  arith_type=Unsigned  n_bits=1  bin_pt=0  preci_type=Single  exp_width=8  frac_width=24  quantization="Round  (unbiased: +/- Inf)"  overflow=Saturate  period=1  dbl_ovrd=off  timing_constraint=None  locs_specified=off  LOCs={}  UseAsADC=off  ADCChannel='1'  inherit_from_input=off  hdl_port=on  block_type=gatewayin
  xps_library_ADCs_adc083000x2_adc1_user_outofrange : xbsIndex_r4/Gateway In  gui_display_data_type=Fixed-point  arith_type=Unsigned  n_bits=4  bin_pt=0  preci_type=Single  exp_width=8  frac_width=24  quantization="Round  (unbiased: +/- Inf)"  overflow=Saturate  period=1  dbl_ovrd=off  timing_constraint=None  locs_specified=off  LOCs={}  UseAsADC=off  ADCChannel='1'  inherit_from_input=off  hdl_port=on  block_type=gatewayin
  xps_library_ADCs_adc083000x2_adc1_user_s{0..7} (8 alike) : xbsIndex_r4/Gateway In  gui_display_data_type=Fixed-point  arith_type=Unsigned  n_bits=8  bin_pt=0  preci_type=Single  exp_width=8  frac_width=24  quantization="Round  (unbiased: +/- Inf)"  overflow=Saturate  period=1  dbl_ovrd=off  timing_constraint=None  locs_specified=off  LOCs={}  UseAsADC=off  ADCChannel='1'  inherit_from_input=off  hdl_port=on  block_type=gatewayin
  xps_library_ADCs_adc083000x2_adc1_user_s0_conv : xps_library/ADCs/conv  bit_width=8
  xps_library_ADCs_adc083000x2_adc1_user_s1_conv : xps_library/ADCs/conv  bit_width=8
  xps_library_ADCs_adc083000x2_adc1_user_s2_conv : xps_library/ADCs/conv  bit_width=8
  xps_library_ADCs_adc083000x2_adc1_user_s3_conv : xps_library/ADCs/conv  bit_width=8
  xps_library_ADCs_adc083000x2_adc1_user_s4_conv : xps_library/ADCs/conv  bit_width=8
  xps_library_ADCs_adc083000x2_adc1_user_s5_conv : xps_library/ADCs/conv  bit_width=8
  xps_library_ADCs_adc083000x2_adc1_user_s6_conv : xps_library/ADCs/conv  bit_width=8
  xps_library_ADCs_adc083000x2_adc1_user_s7_conv : xps_library/ADCs/conv  bit_width=8
  xps_library_ADCs_adc083000x2_adc1_user_sync : xbsIndex_r4/Gateway In  gui_display_data_type=Fixed-point  arith_type=Unsigned  n_bits=4  bin_pt=0  preci_type=Single  exp_width=8  frac_width=24  quantization="Round  (unbiased: +/- Inf)"  overflow=Saturate  period=1  dbl_ovrd=off  timing_constraint=None  locs_specified=off  LOCs={}  UseAsADC=off  ADCChannel='1'  inherit_from_input=off  hdl_port=on  block_type=gatewayin
  adc0_s0 : Outport
  adc1_s0 : Outport  Port=2
  adc0_s1 : Outport  Port=3
  adc1_s1 : Outport  Port=4
  adc0_s2 : Outport  Port=5
  adc1_s2 : Outport  Port=6
  adc0_s3 : Outport  Port=7
  adc1_s3 : Outport  Port=8
  adc0_s4 : Outport  Port=9
  adc1_s4 : Outport  Port=10
  adc0_s5 : Outport  Port=11
  adc1_s5 : Outport  Port=12
  adc0_s6 : Outport  Port=13
  adc1_s6 : Outport  Port=14
  adc0_s7 : Outport  Port=15
  adc1_s7 : Outport  Port=16
  adc0_sync : Outport  Port=17
  adc0_outofrange : Outport  Port=18
  adc0_data_valid : Outport  Port=19
  adc1_sync : Outport  Port=20
  adc1_outofrange : Outport  Port=21
  adc1_data_valid : Outport  Port=22
  wires:
  sim_adc_data_in/1 -> adc_sim/1(sim_adc_data_in)
  adc_sim/1(s0) -> xps_library_ADCs_adc083000x2_adc0_user_s0/1
  xps_library_ADCs_adc083000x2_adc0_user_s0/1 -> xps_library_ADCs_adc083000x2_adc0_user_s0_conv/1
  xps_library_ADCs_adc083000x2_adc0_user_s0_conv/1 -> adc0_s0/1
  adc_sim/2(s1) -> xps_library_ADCs_adc083000x2_adc1_user_s0/1
  xps_library_ADCs_adc083000x2_adc1_user_s0/1 -> xps_library_ADCs_adc083000x2_adc1_user_s0_conv/1
  xps_library_ADCs_adc083000x2_adc1_user_s0_conv/1 -> adc1_s0/1
  adc_sim/3(s2) -> xps_library_ADCs_adc083000x2_adc0_user_s1/1
  xps_library_ADCs_adc083000x2_adc0_user_s1/1 -> xps_library_ADCs_adc083000x2_adc0_user_s1_conv/1
  xps_library_ADCs_adc083000x2_adc0_user_s1_conv/1 -> adc0_s1/1
  adc_sim/4(s3) -> xps_library_ADCs_adc083000x2_adc1_user_s1/1
  xps_library_ADCs_adc083000x2_adc1_user_s1/1 -> xps_library_ADCs_adc083000x2_adc1_user_s1_conv/1
  xps_library_ADCs_adc083000x2_adc1_user_s1_conv/1 -> adc1_s1/1
  adc_sim/5(s4) -> xps_library_ADCs_adc083000x2_adc0_user_s2/1
  xps_library_ADCs_adc083000x2_adc0_user_s2/1 -> xps_library_ADCs_adc083000x2_adc0_user_s2_conv/1
  xps_library_ADCs_adc083000x2_adc0_user_s2_conv/1 -> adc0_s2/1
  adc_sim/6(s5) -> xps_library_ADCs_adc083000x2_adc1_user_s2/1
  xps_library_ADCs_adc083000x2_adc1_user_s2/1 -> xps_library_ADCs_adc083000x2_adc1_user_s2_conv/1
  xps_library_ADCs_adc083000x2_adc1_user_s2_conv/1 -> adc1_s2/1
  adc_sim/7(s6) -> xps_library_ADCs_adc083000x2_adc0_user_s3/1
  xps_library_ADCs_adc083000x2_adc0_user_s3/1 -> xps_library_ADCs_adc083000x2_adc0_user_s3_conv/1
  xps_library_ADCs_adc083000x2_adc0_user_s3_conv/1 -> adc0_s3/1
  adc_sim/8(s7) -> xps_library_ADCs_adc083000x2_adc1_user_s3/1
  xps_library_ADCs_adc083000x2_adc1_user_s3/1 -> xps_library_ADCs_adc083000x2_adc1_user_s3_conv/1
  xps_library_ADCs_adc083000x2_adc1_user_s3_conv/1 -> adc1_s3/1
  adc_sim/9(s8) -> xps_library_ADCs_adc083000x2_adc0_user_s4/1
  xps_library_ADCs_adc083000x2_adc0_user_s4/1 -> xps_library_ADCs_adc083000x2_adc0_user_s4_conv/1
  xps_library_ADCs_adc083000x2_adc0_user_s4_conv/1 -> adc0_s4/1
  adc_sim/10(s9) -> xps_library_ADCs_adc083000x2_adc1_user_s4/1
  xps_library_ADCs_adc083000x2_adc1_user_s4/1 -> xps_library_ADCs_adc083000x2_adc1_user_s4_conv/1
  xps_library_ADCs_adc083000x2_adc1_user_s4_conv/1 -> adc1_s4/1
  adc_sim/11(s10) -> xps_library_ADCs_adc083000x2_adc0_user_s5/1
  xps_library_ADCs_adc083000x2_adc0_user_s5/1 -> xps_library_ADCs_adc083000x2_adc0_user_s5_conv/1
  xps_library_ADCs_adc083000x2_adc0_user_s5_conv/1 -> adc0_s5/1
  adc_sim/12(s11) -> xps_library_ADCs_adc083000x2_adc1_user_s5/1
  xps_library_ADCs_adc083000x2_adc1_user_s5/1 -> xps_library_ADCs_adc083000x2_adc1_user_s5_conv/1
  xps_library_ADCs_adc083000x2_adc1_user_s5_conv/1 -> adc1_s5/1
  adc_sim/13(s12) -> xps_library_ADCs_adc083000x2_adc0_user_s6/1
  xps_library_ADCs_adc083000x2_adc0_user_s6/1 -> xps_library_ADCs_adc083000x2_adc0_user_s6_conv/1
  xps_library_ADCs_adc083000x2_adc0_user_s6_conv/1 -> adc0_s6/1
  adc_sim/14(s13) -> xps_library_ADCs_adc083000x2_adc1_user_s6/1
  xps_library_ADCs_adc083000x2_adc1_user_s6/1 -> xps_library_ADCs_adc083000x2_adc1_user_s6_conv/1
  xps_library_ADCs_adc083000x2_adc1_user_s6_conv/1 -> adc1_s6/1
  adc_sim/15(s14) -> xps_library_ADCs_adc083000x2_adc0_user_s7/1
  xps_library_ADCs_adc083000x2_adc0_user_s7/1 -> xps_library_ADCs_adc083000x2_adc0_user_s7_conv/1
  xps_library_ADCs_adc083000x2_adc0_user_s7_conv/1 -> adc0_s7/1
  adc_sim/16(s15) -> xps_library_ADCs_adc083000x2_adc1_user_s7/1
  xps_library_ADCs_adc083000x2_adc1_user_s7/1 -> xps_library_ADCs_adc083000x2_adc1_user_s7_conv/1
  xps_library_ADCs_adc083000x2_adc1_user_s7_conv/1 -> adc1_s7/1
  adc0_sync_sim/1 -> xps_library_ADCs_adc083000x2_adc0_user_sync/1
  xps_library_ADCs_adc083000x2_adc0_user_sync/1 -> adc0_sync/1
  adc_sim/17(of) -> xps_library_ADCs_adc083000x2_adc0_user_outofrange/1, xps_library_ADCs_adc083000x2_adc1_user_outofrange/1
  xps_library_ADCs_adc083000x2_adc0_user_outofrange/1 -> adc0_outofrange/1
  adc0_data_valid_sim/1 -> xps_library_ADCs_adc083000x2_adc0_user_data_valid/1
  xps_library_ADCs_adc083000x2_adc0_user_data_valid/1 -> adc0_data_valid/1
  adc1_sync_sim/1 -> xps_library_ADCs_adc083000x2_adc1_user_sync/1
  xps_library_ADCs_adc083000x2_adc1_user_sync/1 -> adc1_sync/1
  xps_library_ADCs_adc083000x2_adc1_user_outofrange/1 -> adc1_outofrange/1
  adc1_data_valid_sim/1 -> xps_library_ADCs_adc083000x2_adc1_user_data_valid/1
  xps_library_ADCs_adc083000x2_adc1_user_data_valid/1 -> adc1_data_valid/1

== system xps_library/ADCs/adc16x250-8 ==
  a1_sim : Inport
  a2_sim : Inport  Port=2
  a3_sim : Inport  Port=3
  a4_sim : Inport  Port=4
  b1_sim : Inport  Port=5
  b2_sim : Inport  Port=6
  b3_sim : Inport  Port=7
  b4_sim : Inport  Port=8
  c1_sim : Inport  Port=9
  c2_sim : Inport  Port=10
  c3_sim : Inport  Port=11
  c4_sim : Inport  Port=12
  d1_sim : Inport  Port=13
  d2_sim : Inport  Port=14
  d3_sim : Inport  Port=15
  d4_sim : Inport  Port=16
  xps_library_ADCs_adc16x250_8_a{1..4} (4 alike) : xbsIndex_r4/Gateway In  gui_display_data_type=Fixed-point  arith_type="Signed  (2's comp)"  n_bits=8  bin_pt=7  preci_type=Single  exp_width=8  frac_width=24  quantization="Round  (unbiased: +/- Inf)"  overflow=Saturate  period=1  dbl_ovrd=off  timing_constraint=None  locs_specified=off  LOCs={}  UseAsADC=off  ADCChannel='1'  inherit_from_input=off  hdl_port=on  block_type=gatewayin
  xps_library_ADCs_adc16x250_8_b{1..4} (4 alike) : xbsIndex_r4/Gateway In  gui_display_data_type=Fixed-point  arith_type="Signed  (2's comp)"  n_bits=8  bin_pt=7  preci_type=Single  exp_width=8  frac_width=24  quantization="Round  (unbiased: +/- Inf)"  overflow=Saturate  period=1  dbl_ovrd=off  timing_constraint=None  locs_specified=off  LOCs={}  UseAsADC=off  ADCChannel='1'  inherit_from_input=off  hdl_port=on  block_type=gatewayin
  xps_library_ADCs_adc16x250_8_c{1..4} (4 alike) : xbsIndex_r4/Gateway In  gui_display_data_type=Fixed-point  arith_type="Signed  (2's comp)"  n_bits=8  bin_pt=7  preci_type=Single  exp_width=8  frac_width=24  quantization="Round  (unbiased: +/- Inf)"  overflow=Saturate  period=1  dbl_ovrd=off  timing_constraint=None  locs_specified=off  LOCs={}  UseAsADC=off  ADCChannel='1'  inherit_from_input=off  hdl_port=on  block_type=gatewayin
  xps_library_ADCs_adc16x250_8_d{1..4} (4 alike) : xbsIndex_r4/Gateway In  gui_display_data_type=Fixed-point  arith_type="Signed  (2's comp)"  n_bits=8  bin_pt=7  preci_type=Single  exp_width=8  frac_width=24  quantization="Round  (unbiased: +/- Inf)"  overflow=Saturate  period=1  dbl_ovrd=off  timing_constraint=None  locs_specified=off  LOCs={}  UseAsADC=off  ADCChannel='1'  inherit_from_input=off  hdl_port=on  block_type=gatewayin
  a1 : Outport
  a2 : Outport  Port=2
  a3 : Outport  Port=3
  a4 : Outport  Port=4
  b1 : Outport  Port=5
  b2 : Outport  Port=6
  b3 : Outport  Port=7
  b4 : Outport  Port=8
  c1 : Outport  Port=9
  c2 : Outport  Port=10
  c3 : Outport  Port=11
  c4 : Outport  Port=12
  d1 : Outport  Port=13
  d2 : Outport  Port=14
  d3 : Outport  Port=15
  d4 : Outport  Port=16
  wires:
  a1_sim/1 -> xps_library_ADCs_adc16x250_8_a1/1
  xps_library_ADCs_adc16x250_8_a1/1 -> a1/1  "a1"
  a2_sim/1 -> xps_library_ADCs_adc16x250_8_a2/1
  xps_library_ADCs_adc16x250_8_a2/1 -> a2/1  "a2"
  a3_sim/1 -> xps_library_ADCs_adc16x250_8_a3/1
  xps_library_ADCs_adc16x250_8_a3/1 -> a3/1  "a3"
  a4_sim/1 -> xps_library_ADCs_adc16x250_8_a4/1
  xps_library_ADCs_adc16x250_8_a4/1 -> a4/1  "a4"
  b1_sim/1 -> xps_library_ADCs_adc16x250_8_b1/1
  xps_library_ADCs_adc16x250_8_b1/1 -> b1/1  "b1"
  b2_sim/1 -> xps_library_ADCs_adc16x250_8_b2/1
  xps_library_ADCs_adc16x250_8_b2/1 -> b2/1  "b2"
  b3_sim/1 -> xps_library_ADCs_adc16x250_8_b3/1
  xps_library_ADCs_adc16x250_8_b3/1 -> b3/1  "b3"
  b4_sim/1 -> xps_library_ADCs_adc16x250_8_b4/1
  xps_library_ADCs_adc16x250_8_b4/1 -> b4/1  "b4"
  c1_sim/1 -> xps_library_ADCs_adc16x250_8_c1/1
  xps_library_ADCs_adc16x250_8_c1/1 -> c1/1  "c1"
  c2_sim/1 -> xps_library_ADCs_adc16x250_8_c2/1
  xps_library_ADCs_adc16x250_8_c2/1 -> c2/1  "c2"
  c3_sim/1 -> xps_library_ADCs_adc16x250_8_c3/1
  xps_library_ADCs_adc16x250_8_c3/1 -> c3/1  "c3"
  c4_sim/1 -> xps_library_ADCs_adc16x250_8_c4/1
  xps_library_ADCs_adc16x250_8_c4/1 -> c4/1  "c4"
  d1_sim/1 -> xps_library_ADCs_adc16x250_8_d1/1
  xps_library_ADCs_adc16x250_8_d1/1 -> d1/1  "d1"
  d2_sim/1 -> xps_library_ADCs_adc16x250_8_d2/1
  xps_library_ADCs_adc16x250_8_d2/1 -> d2/1  "d2"
  d3_sim/1 -> xps_library_ADCs_adc16x250_8_d3/1
  xps_library_ADCs_adc16x250_8_d3/1 -> d3/1  "d3"
  d4_sim/1 -> xps_library_ADCs_adc16x250_8_d4/1
  xps_library_ADCs_adc16x250_8_d4/1 -> d4/1  "d4"
